simulink model "zitaijiao"  (Simulink 5.0)
settings: Solver=ode45  SolverMode=SingleTasking  StartTime=0.0  StopTime=2.0  FixedStep=0.01  RelTol=1e-3
libraries: cstblocks x2, simulink_extras x1
settings Model: LastModifiedBy=Administrator

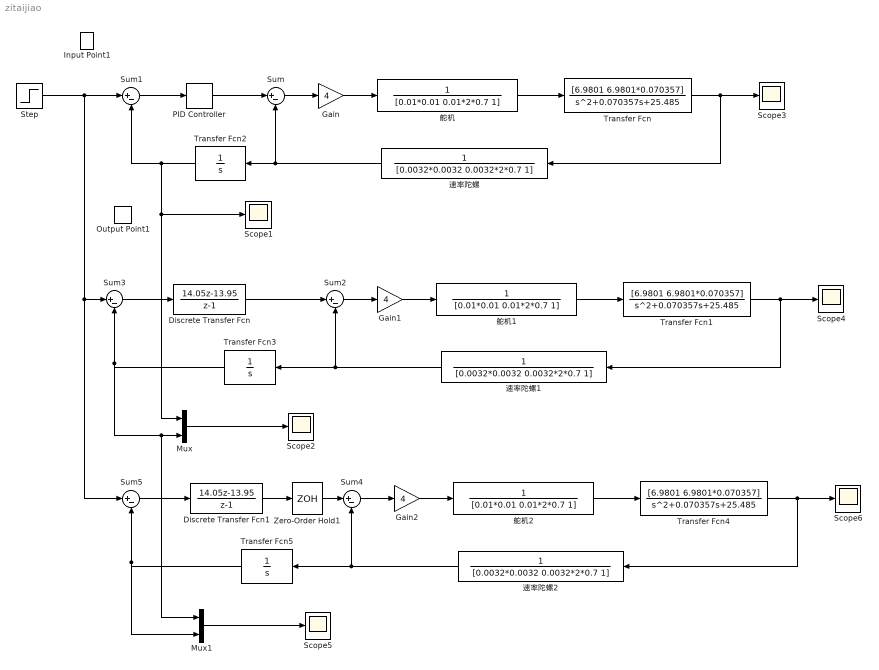
== system zitaijiao ==
  Discrete Transfer Fcn : DiscreteTransferFcn  Numerator=[14.05 -13.95]  Denominator=[1 -1]  SampleTime=0.01
  Discrete Transfer Fcn1 : DiscreteTransferFcn  Numerator=[14.05 -13.95]  Denominator=[1 -1]  SampleTime=0.01
  Gain : Gain  Gain=4  SaturateOnIntegerOverflow=on
  Gain1 : Gain  Gain=4  SaturateOnIntegerOverflow=on
  Gain2 : Gain  Gain=4  SaturateOnIntegerOverflow=on
  Input Point1 : cstblocks/Input Point
  Mux : Mux  Inputs=2
  Mux1 : Mux  Inputs=2
  Output Point1 : cstblocks/Output Point
  PID Controller : simulink_extras/Additional Linear/PID Controller  P=14  I=10  D=0
  Scope{1..6} (6 alike) : Scope
      Scope1 settings: TimeRange=0.8000000000000002  YMin=0.202857  YMax=0.762857  SaveName=alpha  DataFormat=Array
      Scope2 settings: TimeRange=0.8000000000000002  YMin=0.202857  YMax=0.762857  SaveName=alpha1  DataFormat=Array
      Scope3 settings: SaveName=ScopeData2
      Scope5 settings: TimeRange=0.8000000000000002  YMin=0.202857  YMax=0.762857  SaveName=alpha2  DataFormat=Array
  Step : Step  Time=0  SampleTime=0
  Sum{,1..5} (6 alike) : Sum  Inputs=|+-  SaturateOnIntegerOverflow=on
  Transfer Fcn : TransferFcn  Numerator=[6.9801 6.9801*0.070357]  Denominator="[1  0.070357  25.485]"
  Transfer Fcn1 : TransferFcn  Numerator=[6.9801 6.9801*0.070357]  Denominator="[1  0.070357  25.485]"
  Transfer Fcn2 : TransferFcn  Orientation=left  Denominator=[1 0]
  Transfer Fcn3 : TransferFcn  Orientation=left  Denominator=[1 0]
  Transfer Fcn4 : TransferFcn  Numerator=[6.9801 6.9801*0.070357]  Denominator="[1  0.070357  25.485]"
  Transfer Fcn5 : TransferFcn  Orientation=left  Denominator=[1 0]
  Zero-Order Hold1 : ZeroOrderHold  SampleTime=0.01
  舵机 : TransferFcn  Denominator=[0.01*0.01 0.01*2*0.7 1]
  舵机1 : TransferFcn  Denominator=[0.01*0.01 0.01*2*0.7 1]
  舵机2 : TransferFcn  Denominator=[0.01*0.01 0.01*2*0.7 1]
  速率陀螺 : TransferFcn  Orientation=left  Denominator=[0.0032*0.0032 0.0032*2*0.7 1]
  速率陀螺1 : TransferFcn  Orientation=left  Denominator=[0.0032*0.0032 0.0032*2*0.7 1]
  速率陀螺2 : TransferFcn  Orientation=left  Denominator=[0.0032*0.0032 0.0032*2*0.7 1]
  wires:
  舵机/1 -> Transfer Fcn/1
  Gain/1 -> 舵机/1
  Transfer Fcn/1 -> 速率陀螺/1, Scope3/1
  Sum/1 -> Gain/1
  Sum1/1 -> PID Controller/1
  PID Controller/1 -> Sum/1
  Transfer Fcn2/1 -> Sum1/2, Scope1/1, Mux/1
  Step/1 -> Sum1/1, Sum3/1, Sum5/1
  速率陀螺/1 -> Sum/2, Transfer Fcn2/1
  舵机1/1 -> Transfer Fcn1/1
  Gain1/1 -> 舵机1/1
  Transfer Fcn1/1 -> Scope4/1, 速率陀螺1/1
  Sum2/1 -> Gain1/1
  Sum3/1 -> Discrete Transfer Fcn/1
  Discrete Transfer Fcn/1 -> Sum2/1
  Transfer Fcn3/1 -> Sum3/2, Mux/2, Mux1/1
  速率陀螺1/1 -> Transfer Fcn3/1, Sum2/2
  Mux/1 -> Scope2/1
  舵机2/1 -> Transfer Fcn4/1
  Gain2/1 -> 舵机2/1
  Transfer Fcn4/1 -> 速率陀螺2/1, Scope6/1
  Sum4/1 -> Gain2/1
  Sum5/1 -> Discrete Transfer Fcn1/1
  Discrete Transfer Fcn1/1 -> Zero-Order Hold1/1
  Transfer Fcn5/1 -> Mux1/2, Sum5/2
  速率陀螺2/1 -> Sum4/2, Transfer Fcn5/1
  Mux1/1 -> Scope5/1
  Zero-Order Hold1/1 -> Sum4/1
